simulink model "ClusterMG_1_SG"  (R2020a)
settings: Solver=FixedStepAuto  StartTime=0.0  StopTime=Tss  RelTol=1e-5  AbsTol=1e-5  EnableMultiTasking=on
values from neighbouring files (symbols this model uses):
  KA = K_sweep(cont)    [fault_tesis_1_SG.m]
  Ti = 1.5e-4    (= 0.00015)    [fault_tesis_1_SG.m]
  Tof = 1    [fault_tesis_1_SG.m]
undefined symbols (not defined in the file or in its folder): DiscIntNeverNeededParam, sigbuilder_block
libraries: powerlib x88, powerlib_meascontrol x49, simulink x20, spsExcitationSystemModel x1
(part 1 of 3)
settings Model: SimulationMode=accelerator  Creator=GibranZigma  LastModifiedBy=dumay
settings SolverCC: AutoScaleAbsTol=off
settings DataIOCC: Decimation=5  FinalStateName=xss  InitialState=xo  LoadInitialState=on  SaveFinalState=on  SaveFormat=Structure  SaveState=on  ReturnWorkspaceOutputs=off
settings OptimizationCC: LifeSpan=inf
settings DebuggingCC: UnderspecifiedInitializationDetection=Classic  MergeDetectMultiDrivingBlocksExec=none  AllowSymbolicDim=off  StateNameClashWarn=warning  SFUnexpectedBacktrackingDiag=warning  SFNoUnconditionalDefaultTransitionDiag=warning  SFExecutionAtInitializationDiag=none  ArithmeticOperatorsInVariantConditions=warning
settings HardwareCC: ProdBitPerPointer=32  ProdBitPerSizeT=32  ProdBitPerPtrDiffT=32  ProdLargestAtomicFloat=None  ProdIntDivRoundTo=Undefined  ProdEndianess=Unspecified  ProdWordSize=32  ProdHWDeviceType=32-bit Generic
settings ModelReferenceCC: PropagateSignalLabelsOutOfModel=off
settings SFSimCC: SimUseLocalCustomCode=off  CustomCodeUndefinedFunction=UseInterfaceOnly
settings RTWCC: RTWUseLocalCustomCode=off
settings CodeAppCC: StateflowObjectComments=on
settings GRTTargetCC: TargetLangStandard=C89/C90 (ANSI)
settings ConfigComp: CovMetricSettings=dw  CovHtmlReporting=on  CovSaveCumulativeToWorkspaceVar=on  CovSaveSingleToWorkspaceVar=on  CovExternalEMLEnable=off
settings SimscapeCC: SimscapeNormalizeSystem=off

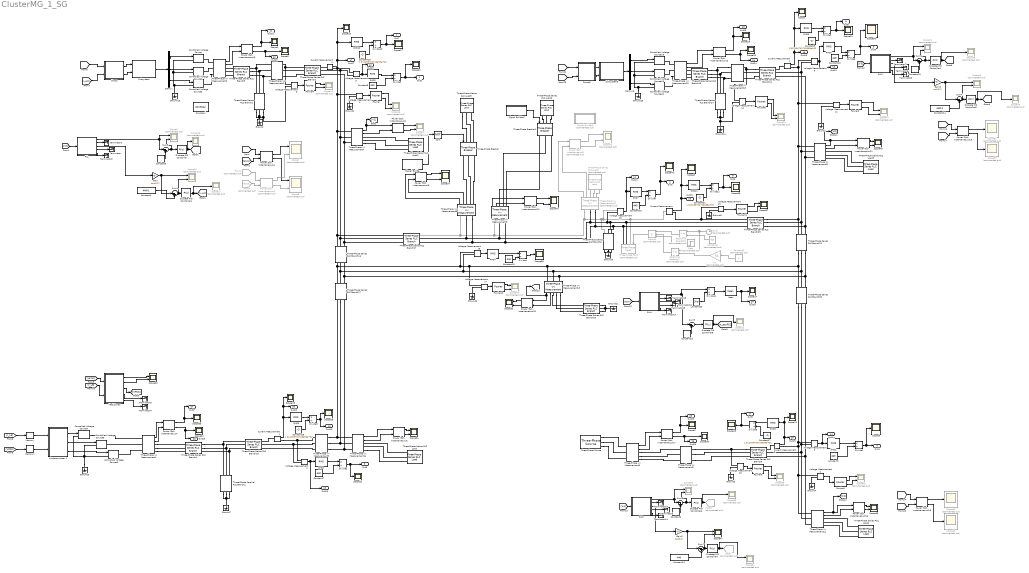
== system ClusterMG_1_SG ==
  Clock : Clock  Commented=on
  Constant{1,7..8,10..11,15..16} (7 alike) : Constant  Value=440
  Constant{3,6,12..13} (4 alike) : Constant  Value=120*pi
  Constant14 : Constant  Value=440*1
  Constant{9,17..19,21} (5 alike) : Constant  Value=1.312159702703695e+02
  Constant2 : Constant  Commented=on  Value=Tof
  Constant20 : Constant  Value=2*pi
  Constant4 : Constant  Value=440*1
  Constant5 : Constant  Commented=on
  Controlled Voltage Source{,2,18..20} (5 alike) : powerlib/Electrical Sources/Controlled Voltage Source  Initialize=on  Source_Type=AC  Amplitude=440*sqrt(2/3)  Phase=0  Frequency=0  Measurements=None
  Controlled Voltage Source1 : powerlib/Electrical Sources/Controlled Voltage Source  Initialize=on  Source_Type=AC  Amplitude=4400*sqrt(2/3)  Phase=0  Frequency=0  Measurements=None
  Controlled Voltage Source4 : powerlib/Electrical Sources/Controlled Voltage Source  Initialize=on  Source_Type=AC  Amplitude=0  Phase=0  Frequency=0  Measurements=None
  Controlled Voltage Source5 : powerlib/Electrical Sources/Controlled Voltage Source  Initialize=on  Source_Type=AC  Amplitude=0  Phase=0  Frequency=0  Measurements=None
  Controlled Voltage Source6 : powerlib/Electrical Sources/Controlled Voltage Source  Initialize=on  Source_Type=AC  Amplitude=0  Phase=0  Frequency=0  Measurements=None
  Current Measurement{,1..4} (5 alike) : powerlib/Measurements/Current Measurement  PhasorSimulation=off  OutputType=Complex  PSBequivalent=0
  Demux : Demux  Outputs=3
  Demux6 : Demux  Outputs=3
  Discrete PID Controller{,4,6,8} (4 alike) : simulink/Continuous/PID Controller  Controller=PI  Form=Parallel  TimeDomain=Discrete-time  UseExternalTs=off  SampleTime=-1  IntegratorMethod=Forward Euler  FilterMethod=Forward Euler  ControllerParametersSource=internal  P=0.02  I=4  D=0  UseFilter=on  N=100  TunerSelectOption=Transfer Function Based (PID Tuner App)  InitialConditionSource=internal  InitialConditionForIntegrator=0  InitialConditionForFilter=0  DifferentiatorICPrevScaledInput=0  ExternalReset=none  TrackingMode=off  Kt=1  LimitOutput=off  UpperSaturationLimit=inf  LowerSaturationLimit=-inf  LinearizeAsGain=off  AntiWindupMode=none  Kb=1  POutMin=[]  POutMax=[]  IOutMin=[]  IOutMax=[]  DOutMin=[]  DOutMax=[]  NOutMin=[]  NOutMax=[]  SumOutMin=[]  SumOutMax=[]  SaturationOutMin=[]  SaturationOutMax=[]  PParamMin=[]  PParamMax=[]  IParamMin=[]  IParamMax=[]  DParamMin=[]  DParamMax=[]  NParamMin=[]  NParamMax=[]  KbParamMin=[]  KbParamMax=[]  KtParamMin=[]  KtParamMax=[]  KbOutMin=[]  KbOutMax=[]  KtOutMin=[]  KtOutMax=[]  IntegratorOutMin=[]  IntegratorOutMax=[]  FilterOutMin=[]  FilterOutMax=[]  SumI1OutMin=[]  SumI1OutMax=[]  SumI2OutMin=[]  SumI2OutMax=[]  SumI3OutMin=[]  SumI3OutMax=[]  SumI4OutMin=[]  SumI4OutMax=[]  SumDOutMin=[]  SumDOutMax=[]  DifferentiatorOutMin=[]  DifferentiatorOutMax=[]  FilterDiffOutCoefMin=[]  FilterDiffOutCoefMax=[]  ReciprocalOutMin=[]  ReciprocalOutMax=[]  SumDenOutMin=[]  SumDenOutMax=[]  SumNumOutMin=[]  SumNumOutMax=[]  DivideOutMin=[]  DivideOutMax=[]  UdiffTsProdOutMin=[]  UdiffTsProdOutMax=[]  NTsProdOutMin=[]  NTsProdOutMax=[]  UintegralTsProdOutMin=[]  UintegralTsProdOutMax=[]  UngainTsProdOutMin=[]  UngainTsProdOutMax=[]  IntegratorContinuousStateAttributes=''  IntegratorStateMustResolveToSignalObject=off  IntegratorRTWStateStorageClass=Auto  FilterContinuousStateAttributes=''  FilterStateMustResolveToSignalObject=off  FilterRTWStateStorageClass=Auto  ParallelPVariant=InternalParameters  IdealPVariant=Disabled  IVariant=InternalParameters  DVariant=Disabled  IntegratorVariant=Discrete  SatVariant=Disabled  AWVariant=Passthrough  PCopyVariant=Disabled  TRVariant=Disabled  FdbkBlocksVariant=Forward  IdealPFdbkVariant=Disabled  SatFdbkVariant=Disabled  DerivativeFilterVariant=Disabled  NVariant=Disabled  NCopyVariant=Disabled_SignalSpec  FilterICVariant=Disabled  IntegratorICVariant=InternalICs  ExternalResetVariant=Disabled  TRSumVariant=Passthrough  SumFdbkVariant=Disabled  SumVariant=Sum_PI  TsampFilterVariant=InternalTs  TsampNgainVariant=Passthrough  TsampIntegralVariant=Passthrough
  Discrete PID Controller1 : simulink/Continuous/PID Controller  Controller=PI  Form=Parallel  TimeDomain=Discrete-time  UseExternalTs=off  SampleTime=-1  IntegratorMethod=Forward Euler  FilterMethod=Forward Euler  ControllerParametersSource=internal  P=.2  I=4  D=0  UseFilter=on  N=100  TunerSelectOption=Transfer Function Based (PID Tuner App)  InitialConditionSource=internal  InitialConditionForIntegrator=0  InitialConditionForFilter=0  DifferentiatorICPrevScaledInput=0  ExternalReset=none  TrackingMode=off  Kt=1  LimitOutput=off  UpperSaturationLimit=inf  LowerSaturationLimit=-inf  LinearizeAsGain=off  AntiWindupMode=none  Kb=1  POutMin=[]  POutMax=[]  IOutMin=[]  IOutMax=[]  DOutMin=[]  DOutMax=[]  NOutMin=[]  NOutMax=[]  SumOutMin=[]  SumOutMax=[]  SaturationOutMin=[]  SaturationOutMax=[]  PParamMin=[]  PParamMax=[]  IParamMin=[]  IParamMax=[]  DParamMin=[]  DParamMax=[]  NParamMin=[]  NParamMax=[]  KbParamMin=[]  KbParamMax=[]  KtParamMin=[]  KtParamMax=[]  KbOutMin=[]  KbOutMax=[]  KtOutMin=[]  KtOutMax=[]  IntegratorOutMin=[]  IntegratorOutMax=[]  FilterOutMin=[]  FilterOutMax=[]  SumI1OutMin=[]  SumI1OutMax=[]  SumI2OutMin=[]  SumI2OutMax=[]  SumI3OutMin=[]  SumI3OutMax=[]  SumI4OutMin=[]  SumI4OutMax=[]  SumDOutMin=[]  SumDOutMax=[]  DifferentiatorOutMin=[]  DifferentiatorOutMax=[]  FilterDiffOutCoefMin=[]  FilterDiffOutCoefMax=[]  ReciprocalOutMin=[]  ReciprocalOutMax=[]  SumDenOutMin=[]  SumDenOutMax=[]  SumNumOutMin=[]  SumNumOutMax=[]  DivideOutMin=[]  DivideOutMax=[]  UdiffTsProdOutMin=[]  UdiffTsProdOutMax=[]  NTsProdOutMin=[]  NTsProdOutMax=[]  UintegralTsProdOutMin=[]  UintegralTsProdOutMax=[]  UngainTsProdOutMin=[]  UngainTsProdOutMax=[]  IntegratorContinuousStateAttributes=''  IntegratorStateMustResolveToSignalObject=off  IntegratorRTWStateStorageClass=Auto  FilterContinuousStateAttributes=''  FilterStateMustResolveToSignalObject=off  FilterRTWStateStorageClass=Auto  ParallelPVariant=InternalParameters  IdealPVariant=Disabled  IVariant=InternalParameters  DVariant=Disabled  IntegratorVariant=Discrete  SatVariant=Disabled  AWVariant=Passthrough  PCopyVariant=Disabled  TRVariant=Disabled  FdbkBlocksVariant=Forward  IdealPFdbkVariant=Disabled  SatFdbkVariant=Disabled  DerivativeFilterVariant=Disabled  NVariant=Disabled  NCopyVariant=Disabled_SignalSpec  FilterICVariant=Disabled  IntegratorICVariant=InternalICs  ExternalResetVariant=Disabled  TRSumVariant=Passthrough  SumFdbkVariant=Disabled  SumVariant=Sum_PI  TsampFilterVariant=InternalTs  TsampNgainVariant=Passthrough  TsampIntegralVariant=Passthrough
  Discrete PID Controller5 : simulink/Continuous/PID Controller  Controller=PI  Form=Parallel  TimeDomain=Discrete-time  UseExternalTs=off  SampleTime=-1  IntegratorMethod=Forward Euler  FilterMethod=Forward Euler  ControllerParametersSource=internal  P=.2  I=4  D=0  UseFilter=on  N=100  TunerSelectOption=Transfer Function Based (PID Tuner App)  InitialConditionSource=internal  InitialConditionForIntegrator=0  InitialConditionForFilter=0  DifferentiatorICPrevScaledInput=0  ExternalReset=none  TrackingMode=off  Kt=1  LimitOutput=off  UpperSaturationLimit=inf  LowerSaturationLimit=-inf  LinearizeAsGain=off  AntiWindupMode=none  Kb=1  POutMin=[]  POutMax=[]  IOutMin=[]  IOutMax=[]  DOutMin=[]  DOutMax=[]  NOutMin=[]  NOutMax=[]  SumOutMin=[]  SumOutMax=[]  SaturationOutMin=[]  SaturationOutMax=[]  PParamMin=[]  PParamMax=[]  IParamMin=[]  IParamMax=[]  DParamMin=[]  DParamMax=[]  NParamMin=[]  NParamMax=[]  KbParamMin=[]  KbParamMax=[]  KtParamMin=[]  KtParamMax=[]  KbOutMin=[]  KbOutMax=[]  KtOutMin=[]  KtOutMax=[]  IntegratorOutMin=[]  IntegratorOutMax=[]  FilterOutMin=[]  FilterOutMax=[]  SumI1OutMin=[]  SumI1OutMax=[]  SumI2OutMin=[]  SumI2OutMax=[]  SumI3OutMin=[]  SumI3OutMax=[]  SumI4OutMin=[]  SumI4OutMax=[]  SumDOutMin=[]  SumDOutMax=[]  DifferentiatorOutMin=[]  DifferentiatorOutMax=[]  FilterDiffOutCoefMin=[]  FilterDiffOutCoefMax=[]  ReciprocalOutMin=[]  ReciprocalOutMax=[]  SumDenOutMin=[]  SumDenOutMax=[]  SumNumOutMin=[]  SumNumOutMax=[]  DivideOutMin=[]  DivideOutMax=[]  UdiffTsProdOutMin=[]  UdiffTsProdOutMax=[]  NTsProdOutMin=[]  NTsProdOutMax=[]  UintegralTsProdOutMin=[]  UintegralTsProdOutMax=[]  UngainTsProdOutMin=[]  UngainTsProdOutMax=[]  IntegratorContinuousStateAttributes=''  IntegratorStateMustResolveToSignalObject=off  IntegratorRTWStateStorageClass=Auto  FilterContinuousStateAttributes=''  FilterStateMustResolveToSignalObject=off  FilterRTWStateStorageClass=Auto  ParallelPVariant=InternalParameters  IdealPVariant=Disabled  IVariant=InternalParameters  DVariant=Disabled  IntegratorVariant=Discrete  SatVariant=Disabled  AWVariant=Passthrough  PCopyVariant=Disabled  TRVariant=Disabled  FdbkBlocksVariant=Forward  IdealPFdbkVariant=Disabled  SatFdbkVariant=Disabled  DerivativeFilterVariant=Disabled  NVariant=Disabled  NCopyVariant=Disabled_SignalSpec  FilterICVariant=Disabled  IntegratorICVariant=InternalICs  ExternalResetVariant=Disabled  TRSumVariant=Passthrough  SumFdbkVariant=Disabled  SumVariant=Sum_PI  TsampFilterVariant=InternalTs  TsampNgainVariant=Passthrough  TsampIntegralVariant=Passthrough
  Discrete PID Controller7 : simulink/Continuous/PID Controller  Controller=PI  Form=Parallel  TimeDomain=Discrete-time  UseExternalTs=off  SampleTime=-1  IntegratorMethod=Forward Euler  FilterMethod=Forward Euler  ControllerParametersSource=internal  P=.2  I=4  D=0  UseFilter=on  N=100  TunerSelectOption=Transfer Function Based (PID Tuner App)  InitialConditionSource=internal  InitialConditionForIntegrator=0  InitialConditionForFilter=0  DifferentiatorICPrevScaledInput=0  ExternalReset=none  TrackingMode=off  Kt=1  LimitOutput=off  UpperSaturationLimit=inf  LowerSaturationLimit=-inf  LinearizeAsGain=off  AntiWindupMode=none  Kb=1  POutMin=[]  POutMax=[]  IOutMin=[]  IOutMax=[]  DOutMin=[]  DOutMax=[]  NOutMin=[]  NOutMax=[]  SumOutMin=[]  SumOutMax=[]  SaturationOutMin=[]  SaturationOutMax=[]  PParamMin=[]  PParamMax=[]  IParamMin=[]  IParamMax=[]  DParamMin=[]  DParamMax=[]  NParamMin=[]  NParamMax=[]  KbParamMin=[]  KbParamMax=[]  KtParamMin=[]  KtParamMax=[]  KbOutMin=[]  KbOutMax=[]  KtOutMin=[]  KtOutMax=[]  IntegratorOutMin=[]  IntegratorOutMax=[]  FilterOutMin=[]  FilterOutMax=[]  SumI1OutMin=[]  SumI1OutMax=[]  SumI2OutMin=[]  SumI2OutMax=[]  SumI3OutMin=[]  SumI3OutMax=[]  SumI4OutMin=[]  SumI4OutMax=[]  SumDOutMin=[]  SumDOutMax=[]  DifferentiatorOutMin=[]  DifferentiatorOutMax=[]  FilterDiffOutCoefMin=[]  FilterDiffOutCoefMax=[]  ReciprocalOutMin=[]  ReciprocalOutMax=[]  SumDenOutMin=[]  SumDenOutMax=[]  SumNumOutMin=[]  SumNumOutMax=[]  DivideOutMin=[]  DivideOutMax=[]  UdiffTsProdOutMin=[]  UdiffTsProdOutMax=[]  NTsProdOutMin=[]  NTsProdOutMax=[]  UintegralTsProdOutMin=[]  UintegralTsProdOutMax=[]  UngainTsProdOutMin=[]  UngainTsProdOutMax=[]  IntegratorContinuousStateAttributes=''  IntegratorStateMustResolveToSignalObject=off  IntegratorRTWStateStorageClass=Auto  FilterContinuousStateAttributes=''  FilterStateMustResolveToSignalObject=off  FilterRTWStateStorageClass=Auto  ParallelPVariant=InternalParameters  IdealPVariant=Disabled  IVariant=InternalParameters  DVariant=Disabled  IntegratorVariant=Discrete  SatVariant=Disabled  AWVariant=Passthrough  PCopyVariant=Disabled  TRVariant=Disabled  FdbkBlocksVariant=Forward  IdealPFdbkVariant=Disabled  SatFdbkVariant=Disabled  DerivativeFilterVariant=Disabled  NVariant=Disabled  NCopyVariant=Disabled_SignalSpec  FilterICVariant=Disabled  IntegratorICVariant=InternalICs  ExternalResetVariant=Disabled  TRSumVariant=Passthrough  SumFdbkVariant=Disabled  SumVariant=Sum_PI  TsampFilterVariant=InternalTs  TsampNgainVariant=Passthrough  TsampIntegralVariant=Passthrough
  Divide{1..12} (12 alike) : Product  Inputs=*/
  Droop : Subsystem
  Droop6 : Subsystem
  Fourier{,2..4,6,9..11} (8 alike) : powerlib_meascontrol/Measurements/Fourier  Freq=60  n=1  InInit=[0, 0]  Ts=Ti
  From2 : From  Commented=on  GotoTag=Vabc2
  From3 : From  Commented=on  GotoTag=Iabc2
  Gain : Gain  Gain=sqrt(3/2)
  Gain2 : Gain  Gain=sqrt(3/2)
  Gain3 : Gain  Gain=sqrt(3/2)
  Goto7 : Goto  Commented=on  GotoTag=v_pcc4
  Goto8 : Goto  Commented=on  GotoTag=w_pcc4
  Ground{,1..11,14..15} (14 alike) : powerlib/Elements/Ground  LConnTagsString=a
  KA : Gain  Commented=on  Gain=KA
  Mean : powerlib_meascontrol/Measurements/Mean  Freq=60  Vinit=0  Ts=Ti
  Mediciones : Subsystem
  Memory : Memory  InitialCondition=[1.756868404921341e+02 -1.613826034273587e+02 14.304237072354686]
  Memory1 : Memory  InitialCondition=0.987801017545438
  NOT : Logic  Operator=NOT  IconShape=distinctive  AllPortsSameDT=off  OutDataTypeStr=boolean
  PLL : Subsystem
  PLL2 : Subsystem
  PLL3 : Subsystem
  PLL4 : Subsystem
  Power (3ph, Instantaneous){1..4,7..8,10..13,16..18,21} (14 alike) : powerlib_meascontrol/Measurements/Power (3ph, Instantaneous)
  "Power (3ph, Instantaneous)5" : powerlib_meascontrol/Measurements/Power (3ph, Instantaneous)  Commented=on
  "Power (3ph, Instantaneous)6" : powerlib_meascontrol/Measurements/Power (3ph, Instantaneous)  Commented=on
  Product : Product  Commented=on  Inputs=3
  RMS{1,5..11} (8 alike) : powerlib_meascontrol/Measurements/RMS  TrueRMS=on  Freq=60  RMSInit=120  Ts=Ti
  RMS2 : powerlib_meascontrol/Measurements/RMS  TrueRMS=on  Freq=60  RMSInit=0  Ts=Ti
  RMS3 : powerlib_meascontrol/Measurements/RMS  TrueRMS=on  Freq=60  RMSInit=0  Ts=Ti
  RMS4 : powerlib_meascontrol/Measurements/RMS  TrueRMS=on  Freq=60  RMSInit=0  Ts=Ti
  Relational Operator1 : RelationalOperator  Commented=on  Operator=<=  OutDataTypeStr=boolean  RndMeth=Simplest
  Relational Operator2 : RelationalOperator  Commented=on  OutDataTypeStr=boolean  RndMeth=Simplest
  Scope{,1..3,5,9..11,14,19,21..22,24..30,33..35,38,42,50} (25 alike) : Scope
  Scope{12,17..18,45..46,52..53,55,59..60} (10 alike) : Scope  Commented=on
  Scope{4,6..8,13,15..16,23,36,40..41,43..44,48,51,54,58} (17 alike) : Scope  Commented=on  NumInputPorts=2
  Scope{20,31..32,37,47,49,56..57,70} (9 alike) : Scope  NumInputPorts=2
  Signal Builder : Subsystem  Tag=STV Subsys  LoadFcn=sigbuilder_block('load');  StartFcn=sigbuilder_block('start');  StopFcn=sigbuilder_block('stop');  ClipboardFcn=sigbuilder_block('clipboard');  mask(Sigbuilder block){tuvar=[0:10]}
      mask help: Simulink:masks:SigbuilderBlock_MD
      mask init:
      | if ~strcmp(get_param(bdroot(gcbh),'SimulationStatus'),'stopped') tuvar = sigbuilder_block('maskInit'); end
      settings: CopyFcn=sigbuilder_block('copy');  DeleteFcn=sigbuilder_block('delete');  ModelCloseFcn=sigbuilder_block('modelClose');  PreSaveFcn=sigbuilder_block('preSave');  PauseFcn=sigbuilder_block('pause');  ContinueFcn=sigbuilder_block('continue');  NameChangeFcn=sigbuilder_block('namechange');  OpenFcn=sigbuilder_block('open',[404 117.5 550.5 362.5 ]);  CloseFcn=sigbuilder_block('close');
      mask Display: plot(0, 0, 100, 100,[2, 2, 32, 32, 2], [68, 8, 8, 68, 68],[32, 2], [38, 38], [32, 19, 2],[53, 60, 44], [32, 17, 17, 2],[16, 16, 31, 31]);txt = getActiveGroup(gcbh);text(2, 100, txt,'verticalAlignment', 'top');
  Signal Builder1 : Subsystem  Tag=STV Subsys  Commented=on  LoadFcn=sigbuilder_block('load');  StartFcn=sigbuilder_block('start');  StopFcn=sigbuilder_block('stop');  ClipboardFcn=sigbuilder_block('clipboard');  mask(Sigbuilder block){tuvar=[0:10]}
      mask help: Simulink:masks:SigbuilderBlock_MD
      mask init:
      | if ~strcmp(get_param(bdroot(gcbh),'SimulationStatus'),'stopped') tuvar = sigbuilder_block('maskInit'); end
      settings: CopyFcn=sigbuilder_block('copy');  DeleteFcn=sigbuilder_block('delete');  ModelCloseFcn=sigbuilder_block('modelClose');  PreSaveFcn=sigbuilder_block('preSave');  PauseFcn=sigbuilder_block('pause');  ContinueFcn=sigbuilder_block('continue');  NameChangeFcn=sigbuilder_block('namechange');  OpenFcn=sigbuilder_block('open',[404 117.5 550.5 362.5 ]);  CloseFcn=sigbuilder_block('close');
      mask Display: plot(0, 0, 100, 100,[2, 2, 32, 32, 2], [68, 8, 8, 68, 68],[32, 2], [38, 38], [32, 19, 2],[53, 60, 44], [32, 17, 17, 2],[16, 16, 31, 31]);txt = getActiveGroup(gcbh);text(2, 100, txt,'verticalAlignment', 'top');
  Signal Builder2 : Subsystem  Tag=STV Subsys  LoadFcn=sigbuilder_block('load');  StartFcn=sigbuilder_block('start');  StopFcn=sigbuilder_block('stop');  ClipboardFcn=sigbuilder_block('clipboard');  mask(Sigbuilder block){tuvar=[0:10]}
      mask help: Simulink:masks:SigbuilderBlock_MD
      mask init:
      | if ~strcmp(get_param(bdroot(gcbh),'SimulationStatus'),'stopped') tuvar = sigbuilder_block('maskInit'); end
      settings: CopyFcn=sigbuilder_block('copy');  DeleteFcn=sigbuilder_block('delete');  ModelCloseFcn=sigbuilder_block('modelClose');  PreSaveFcn=sigbuilder_block('preSave');  PauseFcn=sigbuilder_block('pause');  ContinueFcn=sigbuilder_block('continue');  NameChangeFcn=sigbuilder_block('namechange');  OpenFcn=sigbuilder_block('open',[404 117.5 550.5 362.5 ]);  CloseFcn=sigbuilder_block('close');
      mask Display: plot(0, 0, 100, 100,[2, 2, 32, 32, 2], [68, 8, 8, 68, 68],[32, 2], [38, 38], [32, 19, 2],[53, 60, 44], [32, 17, 17, 2],[16, 16, 31, 31]);txt = getActiveGroup(gcbh);text(2, 100, txt,'verticalAlignment', 'top');
  Step : Step  Commented=on  Before=1  SampleTime=0
  Subsystem : Subsystem
  Subsystem6 : Subsystem
  Sum{1,4..9} (7 alike) : Sum  Inputs=|-+
  Terminator{,1..4,6..15} (15 alike) : Terminator
  Three-Phase Parallel RLC Branch2 : powerlib/Elements/Three-Phase Parallel RLC Branch  LConnTagsString=A|B|C  RConnTagsString=A|B|C  BranchType=C  Resistance=100  Inductance=0.2e-3  Capacitance=1.56e-3  Measurements=None
      settings: SourceProductBaseCode=PS
  Three-Phase Series RLC Branch1 : powerlib/Elements/Three-Phase Series RLC Branch  LConnTagsString=A|B|C  RConnTagsString=A|B|C  BranchType=RL  Resistance=0.1/20  Inductance=1.25e-3/20  Capacitance=1e-6  Measurements=Branch currents
  Three-Phase Series RLC Branch16 : powerlib/Elements/Three-Phase Series RLC Branch  LConnTagsString=A|B|C  RConnTagsString=A|B|C  BranchType=RL  Resistance=1.15/20  Inductance=5.12e-3/20  Capacitance=1e-6  Measurements=Branch currents
  Three-Phase Series RLC Branch17 : powerlib/Elements/Three-Phase Series RLC Branch  LConnTagsString=A|B|C  RConnTagsString=A|B|C  BranchType=RL  Resistance=0.33/20  Inductance=7.96e-3/20  Capacitance=1e-6  Measurements=Branch currents
  Three-Phase Series RLC Branch18 : powerlib/Elements/Three-Phase Series RLC Branch  LConnTagsString=A|B|C  RConnTagsString=A|B|C  BranchType=RL  Resistance=0.1/20  Inductance=1.25e-3/20  Capacitance=1e-6  Measurements=None
  Three-Phase Series RLC Branch2 : powerlib/Elements/Three-Phase Series RLC Branch  LConnTagsString=A|B|C  RConnTagsString=A|B|C  BranchType=RC  Resistance=0.1  Inductance=1e-3  Capacitance=27e-6  Measurements=None
  Three-Phase Series RLC Branch21 : powerlib/Elements/Three-Phase Series RLC Branch  LConnTagsString=A|B|C  RConnTagsString=A|B|C  BranchType=RL  Resistance=0.1/20  Inductance=1.25e-3/20  Capacitance=1e-6  Measurements=Branch currents
  Three-Phase Series RLC Branch22 : powerlib/Elements/Three-Phase Series RLC Branch  LConnTagsString=A|B|C  RConnTagsString=A|B|C  BranchType=RL  Resistance=0.19/20  Inductance=4.38e-3/20  Capacitance=1e-6  Measurements=Branch currents
  Three-Phase Series RLC Branch24 : powerlib/Elements/Three-Phase Series RLC Branch  LConnTagsString=A|B|C  RConnTagsString=A|B|C  BranchType=RC  Resistance=0.1  Inductance=1e-3  Capacitance=27e-6  Measurements=None
  Three-Phase Series RLC Branch25 : powerlib/Elements/Three-Phase Series RLC Branch  LConnTagsString=A|B|C  RConnTagsString=A|B|C  BranchType=RL  Resistance=0.1  Inductance=1.8e-3  Capacitance=1e-6  Measurements=None
  Three-Phase Series RLC Branch26 : powerlib/Elements/Three-Phase Series RLC Branch  LConnTagsString=A|B|C  RConnTagsString=A|B|C  BranchType=RL  Resistance=2.316735433958703e+01  Inductance=(1.481980827061777e+01)/(120*pi)  Capacitance=1e-6  Measurements=None
  Three-Phase Series RLC Branch27 : powerlib/Elements/Three-Phase Series RLC Branch  LConnTagsString=A|B|C  RConnTagsString=A|B|C  BranchType=RL  Resistance=0.67/20  Inductance=1.3e-3/20  Capacitance=1e-6  Measurements=Branch currents
  Three-Phase Series RLC Branch29 : powerlib/Elements/Three-Phase Series RLC Branch  LConnTagsString=A|B|C  RConnTagsString=A|B|C  BranchType=RL  Resistance=0.35/20  Inductance=7.7e-3/20  Capacitance=1e-6  Measurements=Branch currents
  Three-Phase Series RLC Branch3 : powerlib/Elements/Three-Phase Series RLC Branch  LConnTagsString=A|B|C  RConnTagsString=A|B|C  BranchType=RL  Resistance=0.1  Inductance=1.8e-3  Capacitance=1e-6  Measurements=None
  Three-Phase Series RLC Branch30 : powerlib/Elements/Three-Phase Series RLC Branch  LConnTagsString=A|B|C  RConnTagsString=A|B|C  BranchType=RL  Resistance=0.75/20  Inductance=2.58e-3/20  Capacitance=1e-6  Measurements=Branch currents
  Three-Phase Series RLC Branch4 : powerlib/Elements/Three-Phase Series RLC Branch  LConnTagsString=A|B|C  RConnTagsString=A|B|C  BranchType=RL  Resistance=0.042  Inductance=0.57e-3  Capacitance=0  Measurements=Branch currents
  Three-Phase Series RLC Branch5 : powerlib/Elements/Three-Phase Series RLC Branch  LConnTagsString=A|B|C  RConnTagsString=A|B|C  BranchType=RL  Resistance=0.1/20  Inductance=1.25e-3/20  Capacitance=1e-6  Measurements=Branch currents
  Three-Phase Series RLC Branch6 : powerlib/Elements/Three-Phase Series RLC Branch  LConnTagsString=A|B|C  RConnTagsString=A|B|C  BranchType=R  Resistance=10000  Inductance=(1.481980827061777e+01)/(120*pi)  Capacitance=1e-6  Measurements=None
  Three-Phase Series RLC Load : powerlib/Elements/Three-Phase Series RLC Load  LConnTagsString=A|B|C  Configuration=Y (grounded)  NominalVoltage=440*1  Vabc=[1e3 1e3 1e3]  Vabcp=[1e3 1e3 1e3]  NominalFrequency=60  UnbalancedPower=off  ActivePower=0.05e6/2  InductivePower=0.15e6/2  CapacitivePower=0  Pabc=[10e3 9e3 11e3]  QLabc=[100 90 110]  QCabc=[100 90 110]  Pabcp=[10e3 9e3 11e3]  QLabcp=[100 90 110]  QCabcp=[100 90 110]  Measurements=None  LoadType=constant Z
  Three-Phase Series RLC Load1 : powerlib/Elements/Three-Phase Series RLC Load  LConnTagsString=A|B|C  Configuration=Y (grounded)  NominalVoltage=440*1  Vabc=[1e3 1e3 1e3]  Vabcp=[1e3 1e3 1e3]  NominalFrequency=60  UnbalancedPower=off  ActivePower=0.2e6/2  InductivePower=0.1e6/2  CapacitivePower=0  Pabc=[10e3 9e3 11e3]  QLabc=[100 90 110]  QCabc=[100 90 110]  Pabcp=[10e3 9e3 11e3]  QLabcp=[100 90 110]  QCabcp=[100 90 110]  Measurements=None  LoadType=constant Z
  Three-Phase Series RLC Load2 : powerlib/Elements/Three-Phase Series RLC Load  Commented=on  LConnTagsString=A|B|C  Configuration=Y (grounded)  NominalVoltage=440*1  Vabc=[1e3 1e3 1e3]  Vabcp=[1e3 1e3 1e3]  NominalFrequency=60  UnbalancedPower=off  ActivePower=0.1e6/2  InductivePower=0.05e6/2  CapacitivePower=0  Pabc=[10e3 9e3 11e3]  QLabc=[100 90 110]  QCabc=[100 90 110]  Pabcp=[10e3 9e3 11e3]  QLabcp=[100 90 110]  QCabcp=[100 90 110]  Measurements=None  LoadType=constant Z
  Three-Phase Series RLC Load3 : powerlib/Elements/Three-Phase Series RLC Load  LConnTagsString=A|B|C  Configuration=Y (grounded)  NominalVoltage=440*1  Vabc=[1e3 1e3 1e3]  Vabcp=[1e3 1e3 1e3]  NominalFrequency=60  UnbalancedPower=off  ActivePower=0.3e6/2  InductivePower=0.25e6/2  CapacitivePower=0  Pabc=[10e3 9e3 11e3]  QLabc=[100 90 110]  QCabc=[100 90 110]  Pabcp=[10e3 9e3 11e3]  QLabcp=[100 90 110]  QCabcp=[100 90 110]  Measurements=None  LoadType=constant Z
  Three-Phase Series RLC Load4 : powerlib/Elements/Three-Phase Series RLC Load  LConnTagsString=A|B|C  Configuration=Y (grounded)  NominalVoltage=440*1.002147205803442  Vabc=[1e3 1e3 1e3]  Vabcp=[1e3 1e3 1e3]  NominalFrequency=60  UnbalancedPower=off  ActivePower=0.2e6/2  InductivePower=0.1e6/2  CapacitivePower=0  Pabc=[10e3 9e3 11e3]  QLabc=[100 90 110]  QCabc=[100 90 110]  Pabcp=[10e3 9e3 11e3]  QLabcp=[100 90 110]  QCabcp=[100 90 110]  Measurements=None  LoadType=constant Z
  Three-Phase Series RLC Load5 : powerlib/Elements/Three-Phase Series RLC Load  LConnTagsString=A|B|C  Configuration=Y (grounded)  NominalVoltage=440*1  Vabc=[1e3 1e3 1e3]  Vabcp=[1e3 1e3 1e3]  NominalFrequency=60  UnbalancedPower=off  ActivePower=0.1e6/2  InductivePower=0.05e6/2  CapacitivePower=0  Pabc=[10e3 9e3 11e3]  QLabc=[100 90 110]  QCabc=[100 90 110]  Pabcp=[10e3 9e3 11e3]  QLabcp=[100 90 110]  QCabcp=[100 90 110]  Measurements=None  LoadType=constant Z
  Three-Phase Series RLC Load6 : powerlib/Elements/Three-Phase Series RLC Load  LConnTagsString=A|B|C  Configuration=Y (grounded)  NominalVoltage=440*1  Vabc=[1e3 1e3 1e3]  Vabcp=[1e3 1e3 1e3]  NominalFrequency=60  UnbalancedPower=off  ActivePower=0.1e6/1.5  InductivePower=0.05e6/1.5  CapacitivePower=0  Pabc=[10e3 9e3 11e3]  QLabc=[100 90 110]  QCabc=[100 90 110]  Pabcp=[10e3 9e3 11e3]  QLabcp=[100 90 110]  QCabcp=[100 90 110]  Measurements=None  LoadType=constant Z
  Three-Phase V-I Measurement1 : powerlib/Measurements/Three-Phase V-I Measurement  VoltageMeasurement=phase-to-ground  SetLabelV=on  LabelV=Vabc1  Vpu=off  VpuLL=off  CurrentMeasurement=yes  SetLabelI=on  LabelI=Iabc1  Ipu=off  Pbase=100e6  Vbase=500e3  OutputType=Complex  PhasorSimulation=off  PSBequivalent=0
  Three-Phase V-I Measurement{2,4,6..9,12..14,16,21} (11 alike) : powerlib/Measurements/Three-Phase V-I Measurement  VoltageMeasurement=phase-to-ground  SetLabelV=off  LabelV=Vabc  Vpu=off  VpuLL=off  CurrentMeasurement=yes  SetLabelI=off  LabelI=Iabc  Ipu=off  Pbase=100e6  Vbase=500e3  OutputType=Complex  PhasorSimulation=off  PSBequivalent=0
  Three-Phase V-I Measurement15 : powerlib/Measurements/Three-Phase V-I Measurement  VoltageMeasurement=phase-to-ground  SetLabelV=on  LabelV=Vabc13  Vpu=off  VpuLL=off  CurrentMeasurement=yes  SetLabelI=on  LabelI=Iabc13  Ipu=off  Pbase=100e6  Vbase=500e3  OutputType=Complex  PhasorSimulation=off  PSBequivalent=0
  Three-Phase V-I Measurement17 : powerlib/Measurements/Three-Phase V-I Measurement  Commented=on  VoltageMeasurement=phase-to-ground  SetLabelV=off  LabelV=Vabc  Vpu=off  VpuLL=off  CurrentMeasurement=yes  SetLabelI=off  LabelI=Iabc  Ipu=off  Pbase=100e6  Vbase=500e3  OutputType=Complex  PhasorSimulation=off  PSBequivalent=0
  Three-Phase V-I Measurement3 : powerlib/Measurements/Three-Phase V-I Measurement  VoltageMeasurement=phase-to-ground  SetLabelV=on  LabelV=vsin2  Vpu=off  VpuLL=off  CurrentMeasurement=yes  SetLabelI=on  LabelI=I_L3  Ipu=off  Pbase=100e6  Vbase=500e3  OutputType=Complex  PhasorSimulation=off  PSBequivalent=0
  Three-Phase V-I Measurement5 : powerlib/Measurements/Three-Phase V-I Measurement  VoltageMeasurement=phase-to-ground  SetLabelV=on  LabelV=Vabc14  Vpu=off  VpuLL=off  CurrentMeasurement=yes  SetLabelI=on  LabelI=Iabc14  Ipu=off  Pbase=100e6  Vbase=500e3  OutputType=Complex  PhasorSimulation=off  PSBequivalent=0
  Three-Phase Breaker : powerlib/Elements/Three-Phase Breaker  InitialState=closed  SwitchA=on  SwitchB=on  SwitchC=on  SwitchTimes="[1/60  5/60]"  External=on  BreakerResistance=0.01  SnubberResistance=1e6  SnubberCapacitance=inf  Measurements=None
  Three-Phase Breaker1 : powerlib/Elements/Three-Phase Breaker  InitialState=closed  SwitchA=on  SwitchB=on  SwitchC=on  SwitchTimes="[1/60  5/60]"  External=on  BreakerResistance=0.01  SnubberResistance=1e6  SnubberCapacitance=inf  Measurements=None
  Three-Phase Fault : powerlib/Elements/Three-Phase Fault  Commented=on  InitialStates=0  FaultA=on  FaultB=on  FaultC=on  GroundFault=on  SwitchTimes="[1/60  5/60]"  External=on  SwitchStatus=NaN  FaultResistance=0.001  GroundResistance=0.01  SnubberResistance=1e6  SnubberCapacitance=inf  Measurements=None
  Three-Phase Source : powerlib/Electrical Sources/Three-Phase Source  InternalConnection=Yg  VoltagePhases=off  Voltage=440  PhaseAngle=9.121262613448877e+01  Voltage_phases=[25e3 25e3 25e3]/sqrt(3)  PhaseAngles_phases=[0 -120 +120]  Frequency=60  NonIdealSource=on  SpecifyImpedance=off  Resistance=1e-6  Inductance=0  ShortCircuitLevel=100e6  BaseVoltage=25e3  XRratio=7  BusType=swing  Pref=10e3  Qref=0  Prefabc=[10e3, 10e3, 10e3]  Qrefabc=[0, 0, 0]  Qmin=-inf  Qmax=inf
  Voltage Measurement{1..5,8..9,11..12,15..19} (14 alike) : powerlib/Measurements/Voltage Measurement  PhasorSimulation=off  OutputType=Complex  PSBequivalent=0
  powergui : powerlib/powergui  Priority=1  SimulationMode=Discrete  SampleTime=Ti  frequency=60  Iterations=50  frequencyindice=0  Pbase=100e6  ErrMax=1e-4  UnitsV=kV  UnitsW=MW  buscounter=0  FunctionMessages=off  echomessages=off  EnableUseOfTLC=off  CurrentSourceSwitches=off  DisableSnubberDevices=off  DisableRonSwitches=off  DisableVfSwitches=off  DisplayEquations=off  AutomaticDiscreteSolvers=off  SolverType=Tustin  Interpol=off  ExternalGateDelay=off  methode=off  Ts=0  x0status=zero  SPID=off  SwTol=0  HookPort=off  NonlinearTolerance=1e-4  nMaxIteration=100  ContinueOnMaxIteration=off  RestoreLinks=warning  ResistiveCurrentMeasurement=off  Frange=[0:50:15000]  Ylog=off  Xlog=off  ShowGrid=on  save=off  variable=ZData  structure=0  ZoomFFT=off  StartTime=0.0  cycles=1  DisplayStyle=1  fundamental=60  FreqAxis=off  MaxFrequency=1000  frequencyindicesteady=1  RmsSteady=1  display=off
  sincroconverter 1 : Subsystem
  Out1 : Outport
  Out2 : Outport  Port=2
  Out3 : Outport  Port=3
  Out4 : Outport  Port=4
  Out5 : Outport  Port=5
  Out6 : Outport  Port=6
  Out7 : Outport  Port=7
  Out8 : Outport  Port=8
  Out9 : Outport  Port=9
  Out10 : Outport  Port=10
  Out11 : Outport  Port=11
  Out12 : Outport  Port=12
  Out13 : Outport  Port=13
  Out14 : Outport  Port=14
  Out15 : Outport  Port=15
  Out16 : Outport  Port=16
  Out17 : Outport  Port=17
  Out18 : Outport  Port=18
  Out19 : Outport  Port=19
  Out20 : Outport  Port=20
  Out21 : Outport  Port=21
  Out22 : Outport  Port=22
  Out23 : Outport  Port=23
  Out24 : Outport  Port=24
  Out25 : Outport  Port=25
  Out26 : Outport  Port=26
  Out27 : Outport  Port=27
  Out28 : Outport  Port=28
  Out29 : Outport  Port=29
  wires:
  Droop/2(V_ref) -> Subsystem/2(V_ref)
  Droop/1(theta1) -> Subsystem/1(theta1)
  Subsystem/1(Vabc_Controlled) -> Demux/1
  Demux/1 -> Controlled Voltage Source/1
  Demux/2 -> Controlled Voltage Source1/1
  Demux/3 -> Controlled Voltage Source2/1
  Three-Phase V-I Measurement2/1 -> "Power (3ph, Instantaneous)3"/1
  Three-Phase V-I Measurement2/2 -> "Power (3ph, Instantaneous)3"/2
  [Vabc1] -> "Power (3ph, Instantaneous)4"/1
  [Iabc1] -> "Power (3ph, Instantaneous)4"/2
  From2/1 -> "Power (3ph, Instantaneous)5"/1
  From3/1 -> "Power (3ph, Instantaneous)5"/2
  "Power (3ph, Instantaneous)4"/1 -> Scope7/1
  "Power (3ph, Instantaneous)4"/2 -> Scope8/1
  "Power (3ph, Instantaneous)5"/2 -> Scope8/2
  "Power (3ph, Instantaneous)5"/1 -> Scope7/2
  "Power (3ph, Instantaneous)1"/1 -> Scope4/1
  "Power (3ph, Instantaneous)1"/2 -> Scope4/2
  Three-Phase V-I Measurement7/1 -> [V1], "Power (3ph, Instantaneous)1"/1
  Three-Phase V-I Measurement7/2 -> "Power (3ph, Instantaneous)1"/2
  [w_pcc] -> Droop/1(w_PCC)
  Discrete PID Controller/1 -> Scope18/1, [w_pcc]
  PLL/1(w) -> Sum5/1, Scope6/1
  Constant3/1 -> Sum5/2
  Sum5/1 -> Discrete PID Controller/1, Scope6/2
  Constant4/1 -> Sum1/2
  Sum1/1 -> Scope15/2, Discrete PID Controller1/1
  Discrete PID Controller1/1 -> Scope17/1, [v_pcc]
  [v_pcc] -> Droop/2(v_PCC)
  Fourier/1 -> Scope16/1
  Fourier/2 -> Scope16/2
  PLL/3(V) -> Gain/1
  PLL/4(vd) -> Terminator/1
  PLL/2(teta) -> Terminator1/1
  PLL/5(vq) -> Terminator2/1
  "Power (3ph, Instantaneous)2"/1 -> Scope31/1
  "Power (3ph, Instantaneous)2"/2 -> Scope31/2
  Three-Phase V-I Measurement14/1 -> "Power (3ph, Instantaneous)2"/1
  Three-Phase V-I Measurement14/2 -> "Power (3ph, Instantaneous)2"/2
  Droop6/2(V_ref) -> Subsystem6/2(V_ref)
  Droop6/1(theta1) -> Subsystem6/1(theta1)
  Subsystem6/1(Vabc_Controlled) -> Demux6/1
  Demux6/1 -> Controlled Voltage Source18/1
  Demux6/2 -> Controlled Voltage Source19/1
  Demux6/3 -> Controlled Voltage Source20/1
  Three-Phase V-I Measurement16/1 -> "Power (3ph, Instantaneous)12"/1
  Three-Phase V-I Measurement16/2 -> "Power (3ph, Instantaneous)12"/2
  [Vabc13] -> "Power (3ph, Instantaneous)13"/1
  [Iabc13] -> "Power (3ph, Instantaneous)13"/2
  "Power (3ph, Instantaneous)13"/1 -> Scope52/1
  "Power (3ph, Instantaneous)13"/2 -> Scope53/1
  "Power (3ph, Instantaneous)11"/1 -> Scope49/1
  "Power (3ph, Instantaneous)11"/2 -> Scope49/2
  Three-Phase V-I Measurement21/1 -> [V3], "Power (3ph, Instantaneous)11"/1
  Three-Phase V-I Measurement21/2 -> "Power (3ph, Instantaneous)11"/2
  [w_pcc3] -> Droop6/1(w_PCC)
  Discrete PID Controller4/1 -> Scope46/1, [w_pcc3]
  PLL2/1(w) -> Sum6/1, Scope51/1
  Constant13/1 -> Sum6/2
  Sum6/1 -> Discrete PID Controller4/1, Scope51/2
  Constant14/1 -> Sum4/2
  Sum4/1 -> Scope43/2, Discrete PID Controller5/1
  Discrete PID Controller5/1 -> Scope45/1, [v_pcc3]
  [v_pcc3] -> Droop6/2(v_PCC)
  Fourier2/1 -> Scope44/1
  Fourier2/2 -> Scope44/2
  PLL2/4(vd) -> Terminator6/1
  PLL2/2(teta) -> Terminator7/1
  PLL2/5(vq) -> Terminator8/1
  Gain/1 -> Sum1/1, Scope15/1
  Gain2/1 -> Sum4/1, Scope43/1
  Three-Phase V-I Measurement6/1 -> "Power (3ph, Instantaneous)17"/1
  Three-Phase V-I Measurement6/2 -> "Power (3ph, Instantaneous)17"/2
  [Vabc14] -> "Power (3ph, Instantaneous)18"/1
  [Iabc14] -> "Power (3ph, Instantaneous)18"/2
  "Power (3ph, Instantaneous)18"/1 -> Scope59/1
  "Power (3ph, Instantaneous)18"/2 -> Scope60/1
  "Power (3ph, Instantaneous)16"/1 -> Scope56/1
  "Power (3ph, Instantaneous)16"/2 -> Scope56/2
  Three-Phase V-I Measurement12/1 -> [V4], "Power (3ph, Instantaneous)16"/1
  Three-Phase V-I Measurement12/2 -> "Power (3ph, Instantaneous)16"/2
  Discrete PID Controller6/1 -> Scope55/1, Goto8/1
  PLL3/1(w) -> Sum8/1, Scope58/1
  Constant6/1 -> Sum8/2
  Sum8/1 -> Discrete PID Controller6/1, Scope58/2
  Constant11/1 -> Sum7/2
  Sum7/1 -> Scope47/2, Discrete PID Controller7/1
  Discrete PID Controller7/1 -> Scope54/1, Goto7/1
  Fourier3/1 -> Scope48/1
  Fourier3/2 -> Scope48/2
  PLL3/4(vd) -> Terminator9/1
  PLL3/2(teta) -> Terminator10/1
  PLL3/5(vq) -> Terminator11/1
  Gain3/1 -> Sum7/1, Scope47/1
  Three-Phase V-I Measurement13/1 -> "Power (3ph, Instantaneous)21"/1, [VCom]
  Three-Phase V-I Measurement13/2 -> "Power (3ph, Instantaneous)21"/2
  "Power (3ph, Instantaneous)21"/1 -> Scope32/1
  "Power (3ph, Instantaneous)21"/2 -> Scope32/2
  Discrete PID Controller8/1 -> Scope12/1, [w_pccPCC]
  PLL4/1(w) -> Divide11/1, Sum9/1
  Constant12/1 -> Sum9/2
  Sum9/1 -> Discrete PID Controller8/1
  PLL4/4(vd) -> Terminator12/1
  PLL4/2(teta) -> Terminator13/1
  PLL4/5(vq) -> Terminator14/1
  Voltage Measurement9/1 -> Fourier4/1
  Fourier4/1 -> Scope13/1
  Fourier4/2 -> Scope13/2
  Voltage Measurement12/1 -> Fourier6/1
  Fourier6/1 -> Scope23/1
  Fourier6/2 -> Scope23/2
  Voltage Measurement15/1 -> Fourier9/1
  Fourier9/2 -> Scope36/2
  Fourier9/1 -> Scope36/1
  Voltage Measurement16/1 -> RMS4/1
  RMS4/1 -> Divide4/1
  Constant15/1 -> Divide4/2
  Divide4/1 -> Scope38/1
  Voltage Measurement17/1 -> Fourier10/1
  Fourier10/1 -> Scope40/1
  Fourier10/2 -> Scope40/2
  Three-Phase V-I Measurement17/1 -> "Power (3ph, Instantaneous)6"/1
  Three-Phase V-I Measurement17/2 -> "Power (3ph, Instantaneous)6"/2
  "Power (3ph, Instantaneous)6"/1 -> Scope41/1
  "Power (3ph, Instantaneous)6"/2 -> Scope41/2
  Voltage Measurement18/1 -> Out11/1, RMS7/1
  RMS7/1 -> Divide7/1
  Constant16/1 -> Divide7/2
  Divide7/1 -> Out1/1, Scope42/1
  Fourier11/1 -> Scope57/1
  Fourier11/2 -> Scope57/2
  Voltage Measurement19/1 -> Fourier11/1
  PLL4/3(V) -> Terminator15/1
  Voltage Measurement4/1 -> Fourier/1
  [V1] -> PLL/1(Vabc)
  Voltage Measurement11/1 -> Fourier2/1
  [V3] -> PLL2/1(Vabc)
  PLL2/3(V) -> Gain2/1
  Voltage Measurement1/1 -> Fourier3/1
  [V4] -> PLL3/1(Vabc)
  PLL3/3(V) -> Gain3/1
  [VCom] -> PLL4/1(Vabc)
  Mediciones/2(Q_1) -> Scope20/2
  [vsin2] -> Mediciones/1(V_pcc)
  Mediciones/3(v_pcc_pu) -> [VPCC]
  [I_L3] -> Mediciones/2(I_L)
  [VPCC] -> Memory1/1
  sincroconverter 1/3(V_c) -> Controlled Voltage Source6/1
  sincroconverter 1/2(V_b) -> Controlled Voltage Source5/1
  [I_L3] -> Memory/1
  sincroconverter 1/1(V_a) -> Controlled Voltage Source4/1
  Mediciones/1(P_1) -> Scope20/1
  Mediciones/4(w_pcc_pu) -> Terminator3/1
  Mediciones/5(ROCOF_pu) -> Terminator4/1
  Relational Operator2/1 -> Product/1
  Clock/1 -> Relational Operator1/1, Relational Operator2/1
  KA/1 -> Relational Operator1/2
  Step/1 -> Product/3
  Relational Operator1/1 -> Product/2
  Constant2/1 -> Relational Operator2/2
  Constant5/1 -> KA/1
  Product/1 -> Three-Phase Fault/1
  Current Measurement/1 -> Out16/1, RMS11/1, Scope3/1
  Current Measurement1/1 -> Out18/1, RMS5/1, Scope/1
  Current Measurement2/1 -> Out17/1, RMS10/1, Scope10/1
  Current Measurement3/1 -> Out19/1, RMS8/1, Scope11/1
  Current Measurement4/1 -> RMS9/1, Out20/1, Scope19/1
  Memory/1 -> sincroconverter 1/1(L)
  Memory1/1 -> sincroconverter 1/2(V_pcc)
  Constant1/1 -> Divide1/2
  Divide1/1 -> Out4/1, Scope9/1
  RMS1/1 -> Divide1/1
  Voltage Measurement5/1 -> Out14/1, RMS1/1
  RMS2/1 -> Divide2/1
  Constant7/1 -> Divide2/2
  Divide2/1 -> Out5/1, Scope21/1
  Voltage Measurement2/1 -> Out15/1, RMS2/1
  RMS3/1 -> Divide3/1
  Constant8/1 -> Divide3/2
  Voltage Measurement3/1 -> Out12/1, RMS3/1
  Divide3/1 -> Out2/1, Scope22/1
  Constant10/1 -> Divide6/2
  RMS6/1 -> Divide6/1
  Divide6/1 -> Out3/1, Scope50/1
  Voltage Measurement8/1 -> Out13/1, RMS6/1
  RMS10/1 -> Divide10/1
  Constant19/1 -> Divide10/2
  Divide10/1 -> Out7/1, Scope27/1
  "Power (3ph, Instantaneous)3"/1 -> Out21/1, Scope1/1
  "Power (3ph, Instantaneous)3"/2 -> Out22/1, Scope5/1
  Divide5/1 -> Out8/1, Scope24/1
  RMS5/1 -> Divide5/1
  Constant9/1 -> Divide5/2
  "Power (3ph, Instantaneous)12"/2 -> Out24/1, Scope26/1
  "Power (3ph, Instantaneous)12"/1 -> Out23/1, Scope25/1
  Constant17/1 -> Divide8/2
  RMS8/1 -> Divide8/1
  Divide8/1 -> Out9/1, Scope28/1
  Constant18/1 -> Divide9/2
  RMS9/1 -> Divide9/1
  Divide9/1 -> Out10/1, Scope29/1
  "Power (3ph, Instantaneous)17"/2 -> Out26/1, Scope30/1
  "Power (3ph, Instantaneous)17"/1 -> Out25/1, Scope2/1
  "Power (3ph, Instantaneous)7"/1 -> Out27/1, Scope33/1
  "Power (3ph, Instantaneous)7"/2 -> Out28/1, Scope34/1
  Three-Phase V-I Measurement4/2 -> "Power (3ph, Instantaneous)7"/2
  Three-Phase V-I Measurement4/1 -> "Power (3ph, Instantaneous)7"/1
  Constant20/1 -> Divide11/2
  Mean/1 -> Out29/1, Scope14/1
  Divide11/1 -> Mean/1
  Divide12/1 -> Out6/1, Scope35/1
  RMS11/1 -> Divide12/1
  Constant21/1 -> Divide12/2
  Signal Builder/1(Signal 1) -> NOT/1
  NOT/1 -> Three-Phase Breaker/1
  Three-Phase V-I Measurement8/1 -> "Power (3ph, Instantaneous)8"/1
  Three-Phase V-I Measurement8/2 -> "Power (3ph, Instantaneous)8"/2
  "Power (3ph, Instantaneous)8"/1 -> Scope37/1
  "Power (3ph, Instantaneous)8"/2 -> Scope37/2
  Three-Phase V-I Measurement9/1 -> "Power (3ph, Instantaneous)10"/1
  "Power (3ph, Instantaneous)10"/2 -> Scope70/2
  Three-Phase V-I Measurement9/2 -> "Power (3ph, Instantaneous)10"/2
  "Power (3ph, Instantaneous)10"/1 -> Scope70/1
  Signal Builder2/1(Signal 1) -> Three-Phase Breaker1/1
  connections:
  Ground/LConn1 -- Voltage Measurement9/LConn2 -- Three-Phase Series RLC Branch2/RConn3 -- Three-Phase Series RLC Branch2/RConn1 -- Three-Phase Series RLC Branch2/RConn2
  Three-Phase V-I Measurement1/RConn1 -- Three-Phase Series RLC Branch1/LConn1 -- Voltage Measurement9/LConn1
  Three-Phase V-I Measurement1/RConn2 -- Three-Phase Series RLC Branch1/LConn2
  Three-Phase V-I Measurement1/RConn3 -- Three-Phase Series RLC Branch1/LConn3
  Three-Phase Series RLC Branch2/LConn2 -- Three-Phase V-I Measurement1/LConn2 -- Three-Phase Series RLC Branch3/RConn2
  Three-Phase Series RLC Branch2/LConn1 -- Three-Phase Series RLC Branch3/RConn1 -- Three-Phase V-I Measurement1/LConn1
  Three-Phase Series RLC Branch2/LConn3 -- Three-Phase Series RLC Branch3/RConn3 -- Three-Phase V-I Measurement1/LConn3
  Controlled Voltage Source2/LConn1 -- Controlled Voltage Source/LConn1 -- Controlled Voltage Source1/LConn1 -- Ground10/LConn1
  Three-Phase V-I Measurement2/LConn1 -- Controlled Voltage Source/RConn1
  Three-Phase V-I Measurement2/LConn2 -- Controlled Voltage Source1/RConn1
  Three-Phase V-I Measurement2/LConn3 -- Controlled Voltage Source2/RConn1
  Three-Phase Series RLC Branch16/LConn1 -- Three-Phase Series RLC Branch27/LConn1 -- Current Measurement2/RConn1 -- Voltage Measurement3/LConn1 -- Voltage Measurement4/LConn1 -- Three-Phase V-I Measurement7/LConn1
  Three-Phase Series RLC Branch16/LConn2 -- Three-Phase Series RLC Branch27/LConn2 -- Three-Phase V-I Measurement7/LConn2 -- Voltage Measurement3/LConn2 -- Three-Phase Series RLC Branch1/RConn2
  Three-Phase V-I Measurement7/LConn3 -- Three-Phase Series RLC Branch16/LConn3 -- Three-Phase Series RLC Branch27/LConn3 -- Three-Phase Series RLC Branch1/RConn3
  Three-Phase Series RLC Branch3/LConn1 -- Three-Phase V-I Measurement2/RConn1
  Three-Phase Series RLC Branch3/LConn2 -- Three-Phase V-I Measurement2/RConn2
  Three-Phase Series RLC Branch3/LConn3 -- Three-Phase V-I Measurement2/RConn3
  Three-Phase V-I Measurement7/RConn2 -- Three-Phase Series RLC Load1/LConn2
  Three-Phase V-I Measurement7/RConn3 -- Three-Phase Series RLC Load1/LConn3
  Three-Phase Series RLC Load1/LConn1 -- Three-Phase V-I Measurement7/RConn1
  Three-Phase V-I Measurement14/LConn1 -- Three-Phase V-I Measurement3/RConn1 -- Three-Phase Series RLC Branch17/RConn1
  Three-Phase Series RLC Branch17/RConn2 -- Three-Phase V-I Measurement3/RConn2 -- Three-Phase V-I Measurement14/LConn2
  Three-Phase V-I Measurement14/LConn3 -- Three-Phase V-I Measurement3/RConn3 -- Three-Phase Series RLC Branch17/RConn3
  Three-Phase Series RLC Load/LConn2 -- Three-Phase V-I Measurement14/RConn2
  Three-Phase V-I Measurement14/RConn3 -- Three-Phase Series RLC Load/LConn3
  Three-Phase Series RLC Load/LConn1 -- Three-Phase V-I Measurement14/RConn1
  Three-Phase Series RLC Branch21/LConn1 -- Three-Phase V-I Measurement15/RConn1 -- Voltage Measurement12/LConn1
  Three-Phase V-I Measurement15/RConn2 -- Three-Phase Series RLC Branch21/LConn2
  Three-Phase Series RLC Branch24/LConn2 -- Three-Phase V-I Measurement15/LConn2 -- Three-Phase Series RLC Branch25/RConn2
  Three-Phase V-I Measurement15/LConn1 -- Three-Phase Series RLC Branch24/LConn1 -- Three-Phase Series RLC Branch25/RConn1
  Three-Phase V-I Measurement15/LConn3 -- Three-Phase Series RLC Branch24/LConn3 -- Three-Phase Series RLC Branch25/RConn3
  Ground15/LConn1 -- Controlled Voltage Source20/LConn1 -- Controlled Voltage Source18/LConn1 -- Controlled Voltage Source19/LConn1
  Three-Phase V-I Measurement21/LConn1 -- Voltage Measurement8/LConn1 -- Current Measurement1/RConn1 -- Voltage Measurement11/LConn1 -- Three-Phase Series RLC Branch29/LConn1 -- Three-Phase Series RLC Branch22/LConn1
  Three-Phase V-I Measurement21/LConn2 -- Three-Phase Series RLC Branch29/LConn2 -- Three-Phase Series RLC Branch22/LConn2 -- Voltage Measurement8/LConn2 -- Three-Phase Series RLC Branch21/RConn2
  Three-Phase V-I Measurement21/LConn3 -- Three-Phase Series RLC Branch29/LConn3 -- Three-Phase Series RLC Branch22/LConn3 -- Three-Phase Series RLC Branch21/RConn3
  Three-Phase V-I Measurement16/LConn2 -- Controlled Voltage Source19/RConn1
  Three-Phase V-I Measurement16/LConn1 -- Controlled Voltage Source18/RConn1
  Three-Phase V-I Measurement16/LConn3 -- Controlled Voltage Source20/RConn1
  Three-Phase Series RLC Branch25/LConn1 -- Three-Phase V-I Measurement16/RConn1
  Three-Phase Series RLC Branch25/LConn3 -- Three-Phase V-I Measurement16/RConn3
  Three-Phase Series RLC Branch25/LConn2 -- Three-Phase V-I Measurement16/RConn2
  Three-Phase Series RLC Load3/LConn2 -- Three-Phase V-I Measurement21/RConn2
  Three-Phase Series RLC Load3/LConn3 -- Three-Phase V-I Measurement21/RConn3
  Three-Phase V-I Measurement15/RConn3 -- Three-Phase Series RLC Branch21/LConn3
  Three-Phase Series RLC Load3/LConn1 -- Three-Phase V-I Measurement21/RConn1
  Three-Phase Series RLC Branch5/LConn1 -- Three-Phase V-I Measurement5/RConn1 -- Voltage Measurement15/LConn1
  Three-Phase V-I Measurement5/RConn2 -- Three-Phase Series RLC Branch5/LConn2
  Three-Phase V-I Measurement6/RConn2 -- Three-Phase V-I Measurement5/LConn2
  Three-Phase V-I Measurement6/RConn1 -- Three-Phase V-I Measurement5/LConn1
  Three-Phase V-I Measurement6/RConn3 -- Three-Phase V-I Measurement5/LConn3
  Three-Phase V-I Measurement12/LConn1 -- Voltage Measurement5/LConn1 -- Three-Phase Series RLC Branch30/LConn1 -- Current Measurement3/RConn1 -- Voltage Measurement1/LConn1
  Three-Phase Series RLC Load4/LConn1 -- Three-Phase V-I Measurement12/RConn1
  Three-Phase Series RLC Load4/LConn3 -- Three-Phase V-I Measurement12/RConn3
  Three-Phase Series RLC Load4/LConn2 -- Three-Phase V-I Measurement12/RConn2
  Three-Phase V-I Measurement12/LConn2 -- Voltage Measurement5/LConn2 -- Three-Phase Series RLC Branch30/LConn2 -- Three-Phase Series RLC Branch5/RConn2
  Three-Phase V-I Measurement5/RConn3 -- Three-Phase Series RLC Branch5/LConn3
  Three-Phase V-I Measurement12/LConn3 -- Three-Phase Series RLC Branch30/LConn3 -- Three-Phase Series RLC Branch5/RConn3
  Three-Phase Series RLC Branch17/LConn2 -- Three-Phase Series RLC Branch30/RConn2 -- Three-Phase Series RLC Branch22/RConn2 -- Three-Phase V-I Measurement13/LConn2 -- Voltage Measurement16/LConn2 -- Three-Phase Series RLC Branch16/RConn2
  Three-Phase Series RLC Branch17/LConn1 -- Voltage Measurement17/LConn1 -- Three-Phase Series RLC Branch30/RConn1 -- Three-Phase Series RLC Branch22/RConn1 -- Three-Phase V-I Measurement13/LConn1 -- Voltage Measurement16/LConn1 -- Three-Phase Series RLC Branch16/RConn1
  Three-Phase Series RLC Branch17/LConn3 -- Three-Phase Series RLC Branch30/RConn3 -- Three-Phase Series RLC Branch22/RConn3 -- Three-Phase V-I Measurement13/LConn3 -- Three-Phase Series RLC Branch16/RConn3
  Three-Phase Fault/LConn1 -- Current Measurement/LConn1 -- Three-Phase Series RLC Branch6/LConn1 -- Three-Phase V-I Measurement17/LConn1 -- Three-Phase V-I Measurement8/LConn1 -- Three-Phase Series RLC Branch27/RConn1 -- Three-Phase V-I Measurement9/LConn1 -- Voltage Measurement18/LConn1
  Three-Phase Series RLC Branch29/RConn2 -- Three-Phase Fault/LConn2 -- Voltage Measurement18/LConn2 -- Three-Phase V-I Measurement17/LConn2 -- Three-Phase V-I Measurement9/LConn2 -- Three-Phase V-I Measurement8/LConn2 -- Three-Phase Series RLC Branch27/RConn2 -- Three-Phase Series RLC Branch6/LConn2
  Three-Phase Series RLC Branch29/RConn3 -- Three-Phase Fault/LConn3 -- Three-Phase V-I Measurement17/LConn3 -- Three-Phase V-I Measurement9/LConn3 -- Three-Phase V-I Measurement8/LConn3 -- Three-Phase Series RLC Branch27/RConn3 -- Three-Phase Series RLC Branch6/LConn3
  Three-Phase Series RLC Branch26/LConn1 -- Three-Phase V-I Measurement13/RConn1
  Three-Phase V-I Measurement13/RConn2 -- Three-Phase Series RLC Branch26/LConn2
  Three-Phase V-I Measurement13/RConn3 -- Three-Phase Series RLC Branch26/LConn3
  Three-Phase Source/RConn1 -- Three-Phase V-I Measurement6/LConn1
  Three-Phase Source/RConn2 -- Three-Phase V-I Measurement6/LConn2
  Three-Phase Source/RConn3 -- Three-Phase V-I Measurement6/LConn3
  Three-Phase Series RLC Branch26/RConn3 -- Three-Phase Series RLC Branch26/RConn1 -- Ground11/LConn1 -- Three-Phase Series RLC Branch26/RConn2
  Ground3/LConn1 -- Voltage Measurement15/LConn2
  Three-Phase Series RLC Load2/LConn1 -- Three-Phase V-I Measurement17/RConn1
  Three-Phase V-I Measurement17/RConn2 -- Three-Phase Series RLC Load2/LConn2
  Three-Phase V-I Measurement17/RConn3 -- Three-Phase Series RLC Load2/LConn3
  Voltage Measurement4/LConn2 -- Ground1/LConn1
  Voltage Measurement11/LConn2 -- Ground2/LConn1
  Three-Phase Series RLC Branch24/RConn1 -- Three-Phase Series RLC Branch24/RConn2 -- Voltage Measurement12/LConn2 -- Ground14/LConn1 -- Three-Phase Series RLC Branch24/RConn3
  Voltage Measurement1/LConn2 -- Ground4/LConn1
  Voltage Measurement19/LConn2 -- Ground5/LConn1
  Voltage Measurement17/LConn2 -- Ground6/LConn1
  Three-Phase Parallel RLC Branch2/LConn1 -- Three-Phase Series RLC Branch18/LConn1 -- Three-Phase Series RLC Branch4/RConn1
  Three-Phase Parallel RLC Branch2/RConn3 -- Three-Phase Parallel RLC Branch2/RConn1 -- Three-Phase Parallel RLC Branch2/RConn2 -- Ground7/LConn1
  Three-Phase Series RLC Branch4/RConn3 -- Three-Phase Parallel RLC Branch2/LConn3 -- Three-Phase Series RLC Branch18/LConn3
  Ground8/LConn1 -- Controlled Voltage Source4/LConn1 -- Controlled Voltage Source5/LConn1 -- Controlled Voltage Source6/LConn1
  Three-Phase Parallel RLC Branch2/LConn2 -- Three-Phase Series RLC Branch4/RConn2 -- Three-Phase Series RLC Branch18/LConn2
  Voltage Measurement19/LConn1 -- Current Measurement/RConn1 -- Three-Phase Series RLC Branch29/RConn1
  Current Measurement1/LConn1 -- Three-Phase Series RLC Branch21/RConn1
  Current Measurement2/LConn1 -- Three-Phase Series RLC Branch1/RConn1
  Current Measurement3/LConn1 -- Three-Phase Series RLC Branch5/RConn1
  Current Measurement4/LConn1 -- Three-Phase Series RLC Branch18/RConn1
  Three-Phase Series RLC Branch6/RConn2 -- Three-Phase Series RLC Branch6/RConn3 -- Ground9/LConn1 -- Three-Phase Series RLC Branch6/RConn1
  Current Measurement4/RConn1 -- Voltage Measurement2/LConn1 -- Three-Phase V-I Measurement3/LConn1
  Voltage Measurement2/LConn2 -- Three-Phase V-I Measurement3/LConn2 -- Three-Phase Series RLC Branch18/RConn2
  Three-Phase V-I Measurement3/LConn3 -- Three-Phase Series RLC Branch18/RConn3
  Three-Phase V-I Measurement4/RConn3 -- Three-Phase Series RLC Branch4/LConn3
  Three-Phase V-I Measurement4/RConn2 -- Three-Phase Series RLC Branch4/LConn2
  Three-Phase V-I Measurement4/RConn1 -- Three-Phase Series RLC Branch4/LConn1
  Three-Phase V-I Measurement4/LConn3 -- Controlled Voltage Source6/RConn1
  Three-Phase V-I Measurement4/LConn2 -- Controlled Voltage Source5/RConn1
  Controlled Voltage Source4/RConn1 -- Three-Phase V-I Measurement4/LConn1
  Three-Phase Breaker/LConn2 -- Three-Phase Series RLC Load5/LConn2
  Three-Phase V-I Measurement8/RConn3 -- Three-Phase Breaker/RConn3
  Three-Phase Series RLC Load5/LConn1 -- Three-Phase Breaker/LConn1
  Three-Phase V-I Measurement8/RConn1 -- Three-Phase Breaker/RConn1
  Three-Phase V-I Measurement8/RConn2 -- Three-Phase Breaker/RConn2
  Three-Phase Breaker/LConn3 -- Three-Phase Series RLC Load5/LConn3
  Three-Phase V-I Measurement9/RConn3 -- Three-Phase Breaker1/RConn3
  Three-Phase V-I Measurement9/RConn2 -- Three-Phase Breaker1/RConn2
  Three-Phase V-I Measurement9/RConn1 -- Three-Phase Breaker1/RConn1
  Three-Phase Breaker1/LConn2 -- Three-Phase Series RLC Load6/LConn2
  Three-Phase Series RLC Load6/LConn3 -- Three-Phase Breaker1/LConn3
  Three-Phase Series RLC Load6/LConn1 -- Three-Phase Breaker1/LConn1
